simulink model "UAVBicopterDynamics"  (R2024b)
settings: Solver=VariableStepAuto  StartTime=0.0  StopTime=10  RelTol=1e-3
settings Model: Creator=Lenovo  LastModifiedBy=Asus
settings RTWCC: GPUComputeCapability=3.5

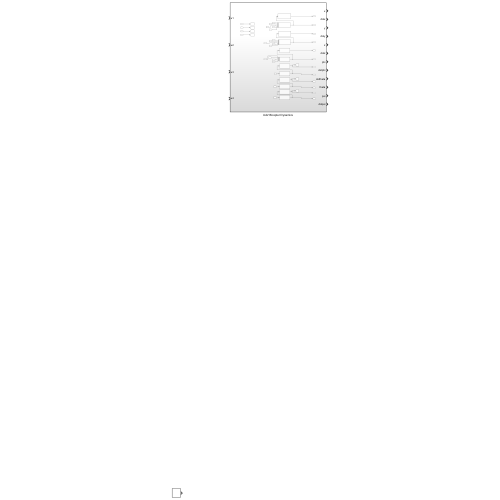
[thumbnail: Simulink's stored preview of the top-level diagram]
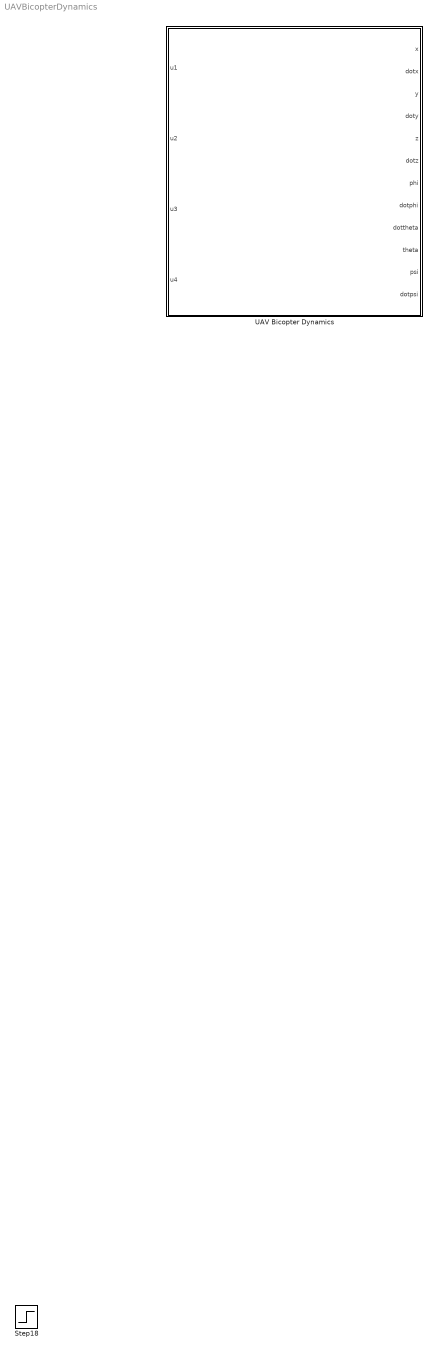
== system UAVBicopterDynamics ==
  Step18 : Step  Time=0  SampleTime=0
  UAV Bicopter Dynamics : Subsystem

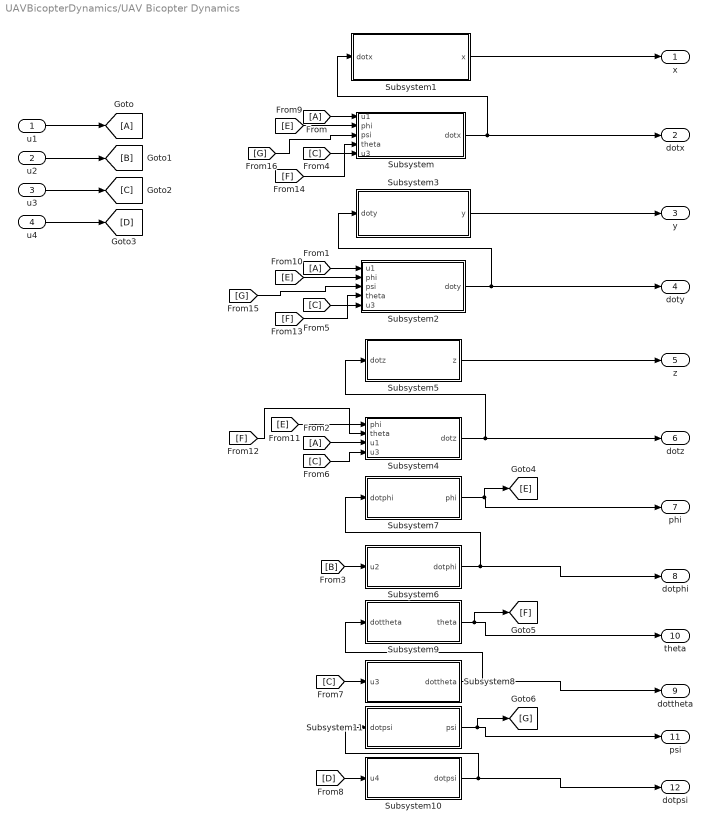
== system UAVBicopterDynamics/UAV Bicopter Dynamics ==
  u1 : Inport
  u2 : Inport  Port=2
  u3 : Inport  Port=3
  u4 : Inport  Port=4
  From : From
  From1 : From
  From2 : From
  Goto : Goto
  Subsystem : Subsystem
  Subsystem1 : Subsystem
  Subsystem10 : Subsystem
  Subsystem11 : Subsystem
  Subsystem2 : Subsystem
  Subsystem3 : Subsystem
  Subsystem4 : Subsystem
  Subsystem5 : Subsystem
  Subsystem6 : Subsystem
  Subsystem7 : Subsystem
  Subsystem8 : Subsystem
  Subsystem9 : Subsystem
  x : Outport
  dotx : Outport  Port=2
  y : Outport  Port=3
  doty : Outport  Port=4
  z : Outport  Port=5
  dotz : Outport  Port=6
  phi : Outport  Port=7
  dotphi : Outport  Port=8
  dottheta : Outport  Port=9
  theta : Outport  Port=10
  psi : Outport  Port=11
  dotpsi : Outport  Port=12
  wires:
  Subsystem/1(dotx) -> Subsystem1/1(dotx), dotx/1
  Subsystem2/1(doty) -> Subsystem3/1(doty), doty/1
  Subsystem4/1(dotz) -> Subsystem5/1(dotz), dotz/1
  Subsystem6/1(dotphi) -> Subsystem7/1(dotphi), dotphi/1
  From/1 -> Subsystem/1(u1)
  From1/1 -> Subsystem2/1(u1)
  From2/1 -> Subsystem4/3(u1)
  [B] -> Subsystem6/1(u2)
  [C] -> Subsystem/5(u3)
  [C] -> Subsystem2/5(u3)
  [C] -> Subsystem4/4(u3)
  [C] -> Subsystem8/1(u3)
  [D] -> Subsystem10/1(u4)
  Subsystem7/1(phi) -> [E], phi/1
  [E] -> Subsystem/2(phi)
  [E] -> Subsystem2/2(phi)
  [E] -> Subsystem4/1(phi)
  [F] -> Subsystem4/2(theta)
  [F] -> Subsystem2/4(theta)
  [F] -> Subsystem/4(theta)
  [G] -> Subsystem2/3(psi)
  [G] -> Subsystem/3(psi)
  Subsystem1/1(x) -> x/1
  Subsystem3/1(y) -> y/1
  Subsystem5/1(z) -> z/1
  u1/1 -> Goto/1
  u2/1 -> [B]
  u3/1 -> [C]
  u4/1 -> [D]
  Subsystem9/1(theta) -> [F], theta/1
  Subsystem8/1(dottheta) -> Subsystem9/1(dottheta), dottheta/1
  Subsystem11/1(psi) -> [G], psi/1
  Subsystem10/1(dotpsi) -> Subsystem11/1(dotpsi), dotpsi/1

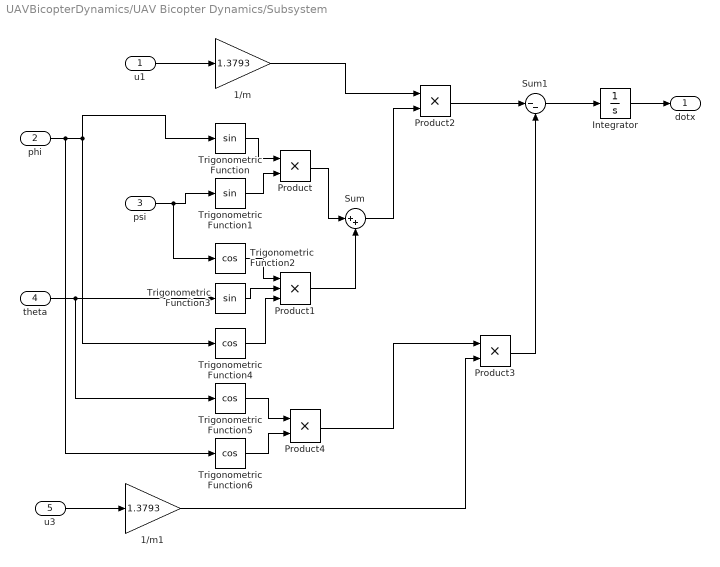
== system UAVBicopterDynamics/UAV Bicopter Dynamics/Subsystem ==
  u1 : Inport
  phi : Inport  Port=2
  psi : Inport  Port=3
  theta : Inport  Port=4
  u3 : Inport  Port=5
  1/m : Gain  Gain=1.3793
  1/m1 : Gain  Gain=1.3793
  Integrator : Integrator
  Product{,2..4} (4 alike) : Product
  Product1 : Product  Inputs=3
  Sum : Sum  Inputs=|++
  Sum1 : Sum  Inputs=|--
  Trigonometric Function : Trigonometry
  Trigonometric Function1 : Trigonometry
  Trigonometric Function{2,4..6} (4 alike) : Trigonometry  Operator=cos
  Trigonometric Function3 : Trigonometry
  dotx : Outport
  wires:
  u1/1 -> 1/m/1
  Trigonometric Function/1 -> Product/1
  Trigonometric Function1/1 -> Product/2
  psi/1 -> Trigonometric Function2/1, Trigonometric Function1/1
  Trigonometric Function2/1 -> Product1/1
  Trigonometric Function3/1 -> Product1/2
  Product/1 -> Sum/1
  1/m/1 -> Product2/1
  Sum/1 -> Product2/2
  Product2/1 -> Sum1/1
  Product1/1 -> Sum/2
  u3/1 -> 1/m1/1
  1/m1/1 -> Product3/2
  Product3/1 -> Sum1/2
  Sum1/1 -> Integrator/1
  Integrator/1 -> dotx/1
  Trigonometric Function4/1 -> Product1/3
  theta/1 -> Trigonometric Function5/1, Trigonometric Function3/1
  phi/1 -> Trigonometric Function6/1, Trigonometric Function4/1, Trigonometric Function/1
  Trigonometric Function5/1 -> Product4/1
  Trigonometric Function6/1 -> Product4/2
  Product4/1 -> Product3/1

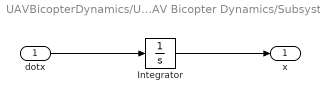
== system UAVBicopterDynamics/UAV Bicopter Dynamics/Subsystem1 ==
  dotx : Inport
  Integrator : Integrator
  x : Outport
  wires:
  dotx/1 -> Integrator/1
  Integrator/1 -> x/1

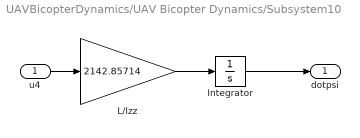
== system UAVBicopterDynamics/UAV Bicopter Dynamics/Subsystem10 ==
  u4 : Inport
  Integrator : Integrator
  L/Izz : Gain  Gain=2142.85714
  dotpsi : Outport
  wires:
  Integrator/1 -> dotpsi/1
  u4/1 -> L/Izz/1
  L/Izz/1 -> Integrator/1

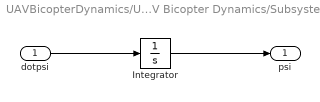
== system UAVBicopterDynamics/UAV Bicopter Dynamics/Subsystem11 ==
  dotpsi : Inport
  Integrator : Integrator
  psi : Outport
  wires:
  Integrator/1 -> psi/1
  dotpsi/1 -> Integrator/1

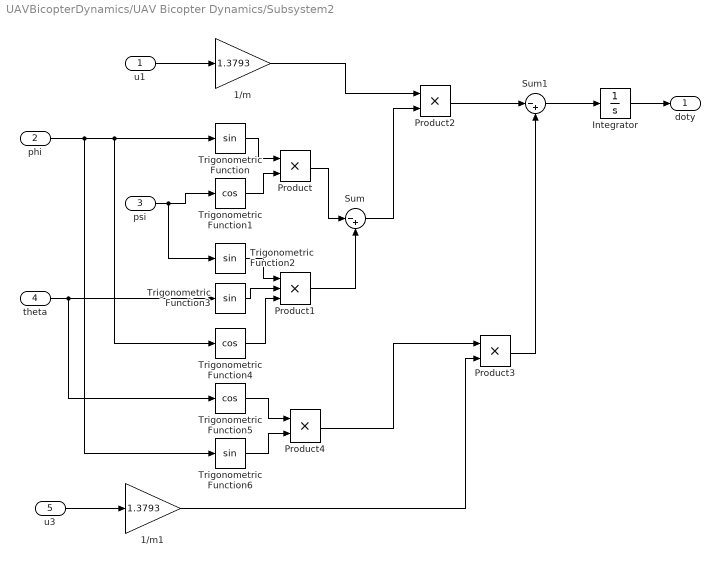
== system UAVBicopterDynamics/UAV Bicopter Dynamics/Subsystem2 ==
  u1 : Inport
  phi : Inport  Port=2
  psi : Inport  Port=3
  theta : Inport  Port=4
  u3 : Inport  Port=5
  1/m : Gain  Gain=1.3793
  1/m1 : Gain  Gain=1.3793
  Integrator : Integrator
  Product{,2..4} (4 alike) : Product
  Product1 : Product  Inputs=3
  Sum : Sum  Inputs=|-+
  Sum1 : Sum  Inputs=|-+
  Trigonometric Function{,2..3,6} (4 alike) : Trigonometry
  Trigonometric Function1 : Trigonometry  Operator=cos
  Trigonometric Function4 : Trigonometry  Operator=cos
  Trigonometric Function5 : Trigonometry  Operator=cos
  doty : Outport
  wires:
  Product1/1 -> Sum/2
  theta/1 -> Trigonometric Function5/1, Trigonometric Function3/1
  Trigonometric Function5/1 -> Product4/1
  Trigonometric Function/1 -> Product/1
  Product4/1 -> Product3/1
  phi/1 -> Trigonometric Function6/1, Trigonometric Function4/1, Trigonometric Function/1
  u3/1 -> 1/m1/1
  psi/1 -> Trigonometric Function2/1, Trigonometric Function1/1
  Sum1/1 -> Integrator/1
  Trigonometric Function4/1 -> Product1/3
  Integrator/1 -> doty/1
  Sum/1 -> Product2/2
  1/m/1 -> Product2/1
  1/m1/1 -> Product3/2
  Trigonometric Function6/1 -> Product4/2
  Product/1 -> Sum/1
  u1/1 -> 1/m/1
  Product2/1 -> Sum1/1
  Trigonometric Function2/1 -> Product1/1
  Trigonometric Function1/1 -> Product/2
  Trigonometric Function3/1 -> Product1/2
  Product3/1 -> Sum1/2

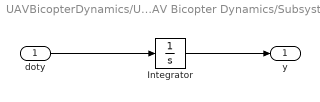
== system UAVBicopterDynamics/UAV Bicopter Dynamics/Subsystem3 ==
  doty : Inport
  Integrator : Integrator
  y : Outport
  wires:
  doty/1 -> Integrator/1
  Integrator/1 -> y/1

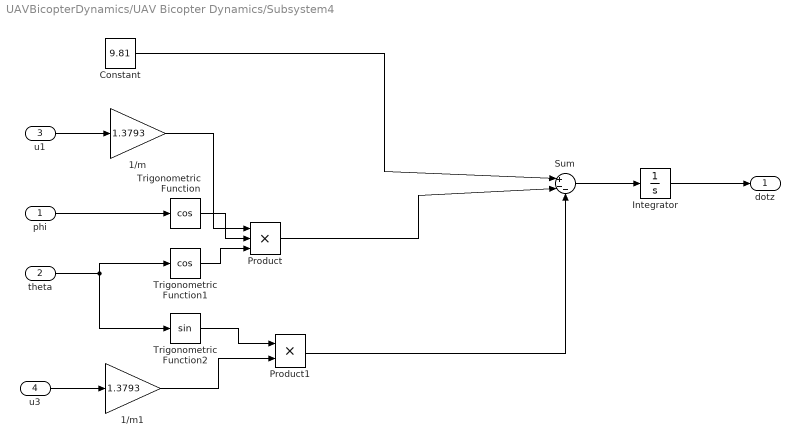
== system UAVBicopterDynamics/UAV Bicopter Dynamics/Subsystem4 ==
  phi : Inport
  theta : Inport  Port=2
  u1 : Inport  Port=3
  u3 : Inport  Port=4
  1/m : Gain  Gain=1.3793
  1/m1 : Gain  Gain=1.3793
  Constant : Constant  Value=9.81
  Integrator : Integrator
  Product : Product  Inputs=3
  Product1 : Product
  Sum : Sum  Inputs=|+--
  Trigonometric Function : Trigonometry  Operator=cos
  Trigonometric Function1 : Trigonometry  Operator=cos
  Trigonometric Function2 : Trigonometry
  dotz : Outport
  wires:
  phi/1 -> Trigonometric Function/1
  1/m/1 -> Product/1
  u1/1 -> 1/m/1
  Trigonometric Function1/1 -> Product/3
  Trigonometric Function/1 -> Product/2
  theta/1 -> Trigonometric Function2/1, Trigonometric Function1/1
  1/m1/1 -> Product1/2
  u3/1 -> 1/m1/1
  Trigonometric Function2/1 -> Product1/1
  Constant/1 -> Sum/1
  Product/1 -> Sum/2
  Product1/1 -> Sum/3
  Sum/1 -> Integrator/1
  Integrator/1 -> dotz/1

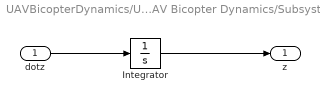
== system UAVBicopterDynamics/UAV Bicopter Dynamics/Subsystem5 ==
  dotz : Inport
  Integrator : Integrator
  z : Outport
  wires:
  dotz/1 -> Integrator/1
  Integrator/1 -> z/1

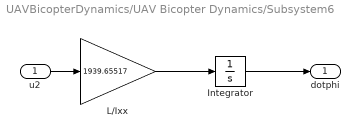
== system UAVBicopterDynamics/UAV Bicopter Dynamics/Subsystem6 ==
  u2 : Inport
  Integrator : Integrator
  L/Ixx : Gain  Gain=1939.65517
  dotphi : Outport
  wires:
  u2/1 -> L/Ixx/1
  L/Ixx/1 -> Integrator/1
  Integrator/1 -> dotphi/1

== system UAVBicopterDynamics/UAV Bicopter Dynamics/Subsystem7 ==
  dotphi : Inport
  Integrator : Integrator
  phi : Outport
  wires:
  dotphi/1 -> Integrator/1
  Integrator/1 -> phi/1

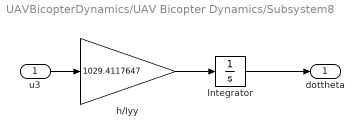
== system UAVBicopterDynamics/UAV Bicopter Dynamics/Subsystem8 ==
  u3 : Inport
  Integrator : Integrator
  h/Iyy : Gain  Gain=1029.4117647
  dottheta : Outport
  wires:
  h/Iyy/1 -> Integrator/1
  Integrator/1 -> dottheta/1
  u3/1 -> h/Iyy/1

== system UAVBicopterDynamics/UAV Bicopter Dynamics/Subsystem9 ==
  dottheta : Inport
  Integrator : Integrator
  theta : Outport
  wires:
  dottheta/1 -> Integrator/1
  Integrator/1 -> theta/1
